simulink model "modelo_dp_completmod"  (Simulink 9.1)
settings: Solver=VariableStepDiscrete  StartTime=0.0  StopTime=sim_time  RelTol=1e-3  EnableMultiTasking=on
values from neighbouring files (symbols this model uses):
  control_fm_am = 1    [configura_modelo_dp_completmod.m]    (also in configura_modulador.m = 0; matlab_WS_mal.mat)
  f_cic_scale = ceil(log2((M*R)^(N-1)))    [conf_mod_filter_design.m]
  fc = 1    [configura_modelo_dp_completmod.m]    (also in configura_modulador.m; matlab_WS_mal.mat)
  fsc = 100    [configura_modelo_dp_completmod.m]    (also in configura_modulador.m; matlab_WS_mal.mat)
  h_comp_cic = round(h_comp_cic*2^16)*2^-16    [conf_mod_filter_design.m]
  h_comp_DAC = round(h_comp_DAC*2^17)*2^-17    [conf_mod_filter_design.m]
  Kfm = 5000    [configura_modelo_dp_completmod.m]    (also in configura_modulador.m; matlab_WS_mal.mat)
  L = 15    [conf_mod_filter_design.m]
  m_am = 1*(1-2^-15)    (= 0.999969482422)    [configura_modelo_dp_completmod.m]    (also in configura_modulador.m; matlab_WS_mal.mat)
  P = round(2^Macc*fmod*1e-3/(fsc/f_interpolacion))*2^-Macc    [conf_mod_filter_design.m]
  R = 2000    [conf_mod_filter_design.m]
  source_sel = 0    [configura_modelo_dp_completmod.m]    (also in configura_modulador.m; matlab_WS_mal.mat = 2)
  W = 16    [conf_mod_filter_design.m]
libraries: dspsigops x6, simulink x2
settings Model: Creator=jvalls  LastModifiedBy=jvalls
settings DataIOCC: LimitDataPoints=on
settings DebuggingCC: UnderspecifiedInitializationDetection=Simplified  MergeDetectMultiDrivingBlocksExec=error  SolverPrmCheckMsg=warning
settings GRTTargetCC: GeneratePreprocessorConditionals=Disable all  CombineOutputUpdateFcns=on  GRTInterface=off
settings ConfigComp: CovSFcnEnable=off

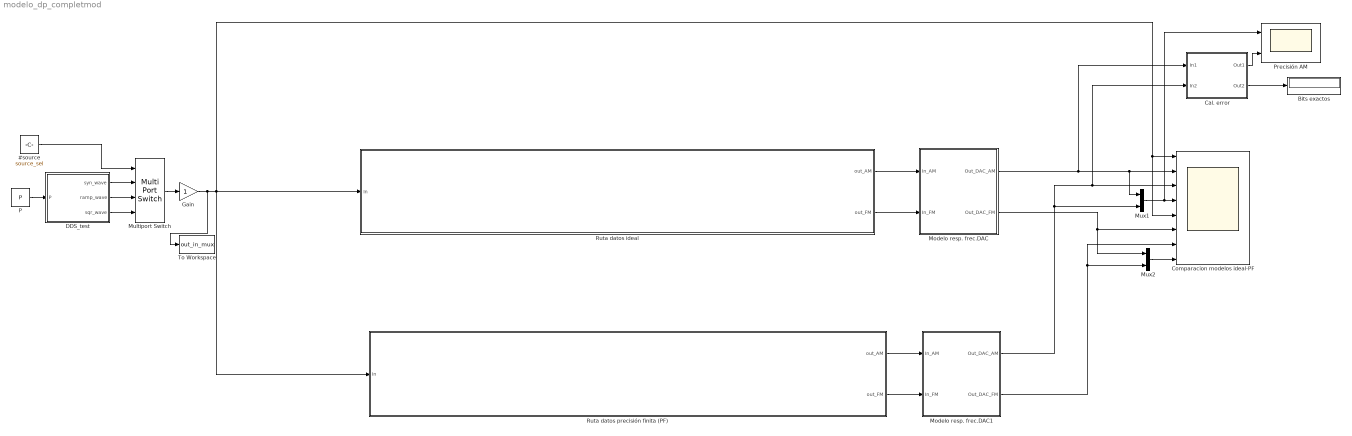
== system modelo_dp_completmod ==
  #source : Constant  Value=source_sel  SampleTime=R/fsc
  Bits exactos : Display
  Cal. error : Subsystem
  Comparacion modelos ideal-PF : Scope  NumInputPorts=8
  DDS_test : Subsystem
  Gain : Gain
  Modelo resp. frec.DAC : Subsystem
  Modelo resp. frec.DAC1 : Subsystem
  Multiport Switch : MultiPortSwitch  DataPortOrder=Specify indices  DataPortIndices={0,1,2}  OutDataTypeStr=double
  Mux1 : Mux  Inputs=2
  Mux2 : Mux  Inputs=2
  P : Constant  Value=P  OutDataTypeStr=fixdt(0,Macc,Macc)  SampleTime=R/fsc
  Precisión AM : Scope  NumInputPorts=2
  Ruta datos ideal : Subsystem
  Ruta datos precisión finita (PF) : Subsystem
  To Workspace : ToWorkspace  VariableName=out_in_mux  SampleTime=-1
      settings: Save2DSignal=2-D array (concatenate along first dimension)
  wires:
  Mux1/1 -> Precisión AM/1, Comparacion modelos ideal-PF/4
  Mux2/1 -> Comparacion modelos ideal-PF/8
  Modelo resp. frec.DAC/1(Out_DAC_AM) -> Cal. error/1(In1), Mux1/1, Comparacion modelos ideal-PF/2
  Modelo resp. frec.DAC1/1(Out_DAC_AM) -> Mux1/2, Cal. error/2(In2), Comparacion modelos ideal-PF/3
  Ruta datos ideal/1(out_AM) -> Modelo resp. frec.DAC/1(In_AM)
  Ruta datos precisión finita (PF)/1(out_AM) -> Modelo resp. frec.DAC1/1(In_AM)
  Ruta datos ideal/2(out_FM) -> Modelo resp. frec.DAC/2(In_FM)
  Ruta datos precisión finita (PF)/2(out_FM) -> Modelo resp. frec.DAC1/2(In_FM)
  Modelo resp. frec.DAC/2(Out_DAC_FM) -> Mux2/1, Comparacion modelos ideal-PF/6
  Modelo resp. frec.DAC1/2(Out_DAC_FM) -> Mux2/2, Comparacion modelos ideal-PF/7
  P/1 -> DDS_test/1(P)
  DDS_test/1(syn_wave) -> Multiport Switch/2
  DDS_test/2(ramp_wave) -> Multiport Switch/3
  DDS_test/3(sqr_wave) -> Multiport Switch/4
  #source/1 -> Multiport Switch/1
  Cal. error/1(Out1) -> Precisión AM/2
  Cal. error/2(Out2) -> Bits exactos/1
  Multiport Switch/1 -> Gain/1
  Gain/1 -> Comparacion modelos ideal-PF/5, Comparacion modelos ideal-PF/1, Ruta datos precisión finita (PF)/1(In), Ruta datos ideal/1(In), To Workspace/1

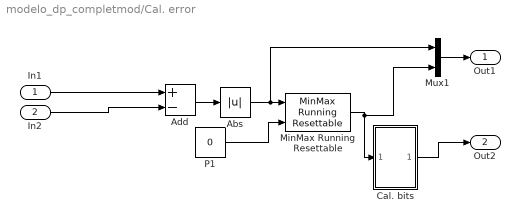
== system modelo_dp_completmod/Cal. error ==
  In1 : Inport
  In2 : Inport  Port=2
  Abs : Abs
  Add : Sum  Inputs=+-
  Cal. bits : Subsystem
  MinMax Running Resettable : simulink/Math Operations/MinMax Running Resettable  Function=max  vinit=0.0
  Mux1 : Mux  Inputs=2
  P1 : Constant  Value=0  OutDataTypeStr=double  SampleTime=-1
  Out1 : Outport
  Out2 : Outport  Port=2
  wires:
  In2/1 -> Add/2
  Abs/1 -> Mux1/1, MinMax Running Resettable/1
  MinMax Running Resettable/1 -> Mux1/2, Cal. bits/1(In1)
  In1/1 -> Add/1
  P1/1 -> MinMax Running Resettable/2
  Add/1 -> Abs/1
  Cal. bits/1(Out1) -> Out2/1
  Mux1/1 -> Out1/1

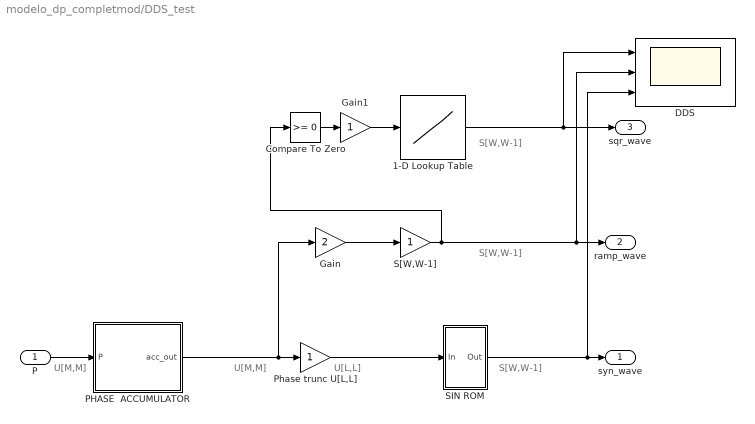
== system modelo_dp_completmod/DDS_test ==
  note: S[W,W-1]
  note: S[W,W-1]
  note: S[W,W-1]
  note: U[M,M]
  note: U[L,L]
  note: U[M,M]
  P : Inport
  1-D Lookup Table : Lookup_n-D  NumberOfTableDimensions=1  BreakpointsForDimension1=[0:1]  Table=[ -1+2^-(W-1) 1-2^-(W-1)]  InternalRulePriority=Speed  RndMeth=Simplest  InputSameDT=on
  Compare To Zero : simulink/Logic and Bit Operations/Compare To Zero  relop=>=  OutDataTypeStr=boolean
  DDS : Scope  NumInputPorts=3
  Gain : Gain  Gain=2  OutDataTypeStr=double
  Gain1 : Gain  OutDataTypeStr=double
  PHASE  ACCUMULATOR : Subsystem
  Phase trunc U[L,L] : Gain  OutDataTypeStr=fixdt(0,L,L)
  SIN ROM : Subsystem
  S[W,W-1] : Gain  OutDataTypeStr=fixdt(1,W,W-1)
  syn_wave : Outport
  ramp_wave : Outport  Port=2
  sqr_wave : Outport  Port=3
  wires:
  Phase trunc U[L,L]/1 -> SIN ROM/1(In)
  SIN ROM/1(Out) -> DDS/3, syn_wave/1
  P/1 -> PHASE  ACCUMULATOR/1(P)
  PHASE  ACCUMULATOR/1(acc_out) -> Phase trunc U[L,L]/1, Gain/1
  Gain1/1 -> 1-D Lookup Table/1
  Compare To Zero/1 -> Gain1/1
  1-D Lookup Table/1 -> sqr_wave/1, DDS/1
  S[W,W-1]/1 -> Compare To Zero/1, DDS/2, ramp_wave/1
  Gain/1 -> S[W,W-1]/1

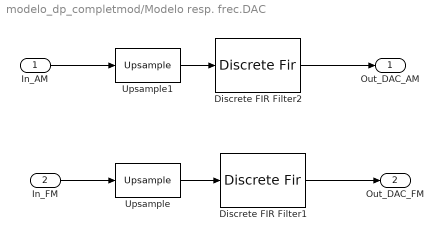
== system modelo_dp_completmod/Modelo resp. frec.DAC ==
  In_AM : Inport
  In_FM : Inport  Port=2
  Discrete FIR Filter1 : DiscreteFir  Coefficients=[1 1 1 1]  InputProcessing=Columns as channels (frame based)
  Discrete FIR Filter2 : DiscreteFir  Coefficients=[1 1 1 1]  InputProcessing=Columns as channels (frame based)
  Upsample : dspsigops/Upsample  N=4  phase=0  InputProcessing=Columns as channels (frame based)  RateOptions=Allow multirate processing  ic=0  mode=Unused parameter value
  Upsample1 : dspsigops/Upsample  N=4  phase=0  InputProcessing=Columns as channels (frame based)  RateOptions=Allow multirate processing  ic=0  mode=Unused parameter value
  Out_DAC_AM : Outport
  Out_DAC_FM : Outport  Port=2
  wires:
  Upsample1/1 -> Discrete FIR Filter2/1
  Upsample/1 -> Discrete FIR Filter1/1
  Discrete FIR Filter2/1 -> Out_DAC_AM/1
  In_AM/1 -> Upsample1/1
  In_FM/1 -> Upsample/1
  Discrete FIR Filter1/1 -> Out_DAC_FM/1

== system modelo_dp_completmod/Modelo resp. frec.DAC1 ==
  In_AM : Inport
  In_FM : Inport  Port=2
  Discrete FIR Filter1 : DiscreteFir  Coefficients=[1 1 1 1]  InputProcessing=Columns as channels (frame based)
  Discrete FIR Filter2 : DiscreteFir  Coefficients=[1 1 1 1]  InputProcessing=Columns as channels (frame based)
  Upsample : dspsigops/Upsample  N=4  phase=0  InputProcessing=Columns as channels (frame based)  RateOptions=Allow multirate processing  ic=0  mode=Unused parameter value
  Upsample1 : dspsigops/Upsample  N=4  phase=0  InputProcessing=Columns as channels (frame based)  RateOptions=Allow multirate processing  ic=0  mode=Unused parameter value
  Out_DAC_AM : Outport
  Out_DAC_FM : Outport  Port=2
  wires:
  Upsample1/1 -> Discrete FIR Filter2/1
  Upsample/1 -> Discrete FIR Filter1/1
  Discrete FIR Filter2/1 -> Out_DAC_AM/1
  In_AM/1 -> Upsample1/1
  In_FM/1 -> Upsample/1
  Discrete FIR Filter1/1 -> Out_DAC_FM/1

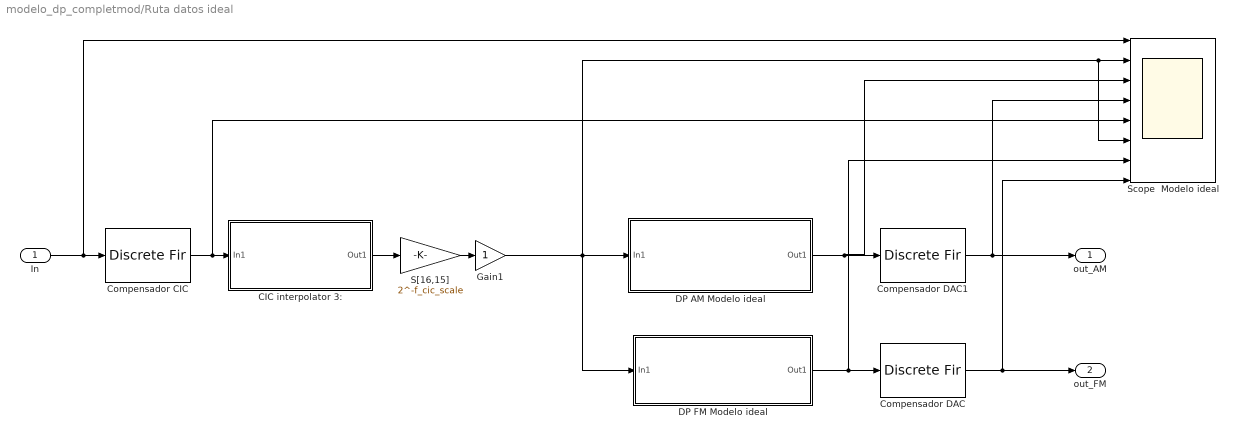
== system modelo_dp_completmod/Ruta datos ideal ==
  In : Inport
  "CIC interpolator 3: " : Subsystem
  Compensador CIC : DiscreteFir  Coefficients=h_comp_cic  InputProcessing=Columns as channels (frame based)
  Compensador DAC : DiscreteFir  Coefficients=h_comp_DAC  InputProcessing=Columns as channels (frame based)
  Compensador DAC1 : DiscreteFir  Coefficients=h_comp_DAC  InputProcessing=Columns as channels (frame based)
  DP AM Modelo ideal : Subsystem
  DP FM Modelo ideal : Subsystem
  Gain1 : Gain  OutDataTypeStr=double
  "S[16,15] " : Gain  Gain=2^-f_cic_scale  OutDataTypeStr=double
  Scope  Modelo ideal : Scope  NumInputPorts=8
  out_AM : Outport
  out_FM : Outport  Port=2
  wires:
  "CIC interpolator 3: "/1(Out1) -> "S[16,15] "/1
  "S[16,15] "/1 -> Gain1/1
  Gain1/1 -> Scope  Modelo ideal/6, Scope  Modelo ideal/2, DP AM Modelo ideal/1(In1), DP FM Modelo ideal/1(In1)
  DP FM Modelo ideal/1(Out1) -> Scope  Modelo ideal/7, Compensador DAC/1
  Compensador DAC/1 -> Scope  Modelo ideal/8, out_FM/1
  Compensador DAC1/1 -> out_AM/1, Scope  Modelo ideal/4
  Compensador CIC/1 -> Scope  Modelo ideal/5, "CIC interpolator 3: "/1(In1)
  DP AM Modelo ideal/1(Out1) -> Scope  Modelo ideal/3, Compensador DAC1/1
  In/1 -> Scope  Modelo ideal/1, Compensador CIC/1

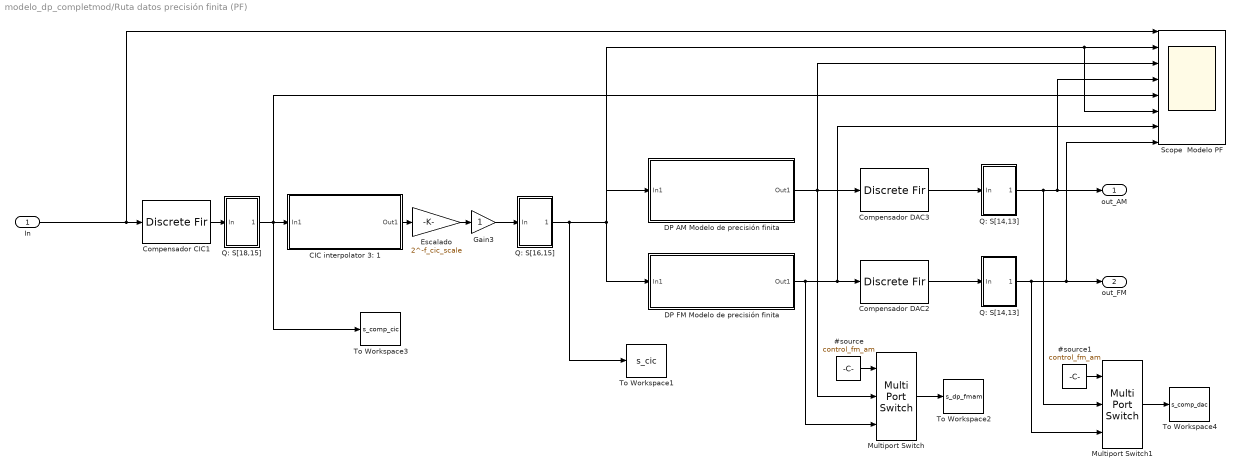
== system modelo_dp_completmod/Ruta datos precisión finita (PF) ==
  In : Inport
  #source : Constant  Value=control_fm_am  SampleTime=1/fsc
  #source1 : Constant  Value=control_fm_am  SampleTime=1/fsc
  CIC interpolator 3: 1 : Subsystem
  Compensador CIC1 : DiscreteFir  Coefficients=h_comp_cic  InputProcessing=Columns as channels (frame based)
  Compensador DAC2 : DiscreteFir  Coefficients=h_comp_DAC  InputProcessing=Columns as channels (frame based)
  Compensador DAC3 : DiscreteFir  Coefficients=h_comp_DAC  InputProcessing=Columns as channels (frame based)
  DP AM Modelo de precisión finita : Subsystem
  DP FM Modelo de precisión finita : Subsystem
  Escalado : Gain  Gain=2^-f_cic_scale  OutDataTypeStr=double
  Gain3 : Gain  OutDataTypeStr=double
  Multiport Switch : MultiPortSwitch  DataPortOrder=Specify indices  DataPortIndices={0,1}  OutDataTypeStr=double
  Multiport Switch1 : MultiPortSwitch  DataPortOrder=Specify indices  DataPortIndices={0,1}  OutDataTypeStr=double
  Q: S[14,13] : Subsystem
  "Q: S[14,13] " : Subsystem
  Q: S[16,15] : Subsystem
  Q: S[18,15] : Subsystem
  Scope  Modelo PF : Scope  NumInputPorts=8
  To Workspace1 : ToWorkspace  VariableName=s_cic  SampleTime=-1
      settings: Save2DSignal=2-D array (concatenate along first dimension)
  To Workspace2 : ToWorkspace  VariableName=s_dp_fmam  SampleTime=-1
      settings: Save2DSignal=2-D array (concatenate along first dimension)
  To Workspace3 : ToWorkspace  VariableName=s_comp_cic  SampleTime=-1
      settings: Save2DSignal=2-D array (concatenate along first dimension)
  To Workspace4 : ToWorkspace  VariableName=s_comp_dac  SampleTime=-1
      settings: Save2DSignal=2-D array (concatenate along first dimension)
  out_AM : Outport
  out_FM : Outport  Port=2
  wires:
  CIC interpolator 3: 1/1(Out1) -> Escalado/1
  Escalado/1 -> Gain3/1
  Compensador CIC1/1 -> Q: S[18,15]/1(In)
  Gain3/1 -> Q: S[16,15]/1(In)
  DP AM Modelo de precisión finita/1(Out1) -> Multiport Switch/2, Scope  Modelo PF/3, Compensador DAC3/1
  Compensador DAC2/1 -> "Q: S[14,13] "/1(In)
  DP FM Modelo de precisión finita/1(Out1) -> Multiport Switch/3, Scope  Modelo PF/7, Compensador DAC2/1
  Compensador DAC3/1 -> Q: S[14,13]/1(In)
  In/1 -> Scope  Modelo PF/1, Compensador CIC1/1
  Q: S[18,15]/1(Out1) -> To Workspace3/1, Scope  Modelo PF/5, CIC interpolator 3: 1/1(In1)
  Q: S[16,15]/1(Out1) -> To Workspace1/1, DP FM Modelo de precisión finita/1(In1), Scope  Modelo PF/6, Scope  Modelo PF/2, DP AM Modelo de precisión finita/1(In1)
  Multiport Switch/1 -> To Workspace2/1
  #source/1 -> Multiport Switch/1
  Q: S[14,13]/1(Out1) -> Multiport Switch1/2, out_AM/1, Scope  Modelo PF/4
  Multiport Switch1/1 -> To Workspace4/1
  #source1/1 -> Multiport Switch1/1
  "Q: S[14,13] "/1(Out1) -> Multiport Switch1/3, Scope  Modelo PF/8, out_FM/1

== system modelo_dp_completmod/Cal. error/Cal. bits ==
  In1 : Inport
  Divide : Product  Inputs=*/
  Math Function : Math  Operator=log10  SaturateOnIntegerOverflow=on
  Math Function1 : Math  Operator=log10  SaturateOnIntegerOverflow=on
  P2 : Constant  Value=2  OutDataTypeStr=double  SampleTime=-1
  Out1 : Outport
  wires:
  P2/1 -> Math Function1/1
  Math Function1/1 -> Divide/2
  In1/1 -> Math Function/1
  Math Function/1 -> Divide/1
  Divide/1 -> Out1/1

== system modelo_dp_completmod/DDS_test/PHASE  ACCUMULATOR ==
  P : Inport
  Add U[M,M] : Sum  AccumDataTypeStr=fixdt(0,Macc,Macc)  OutDataTypeStr=fixdt(0,24,24)  RndMeth=Convergent
  Delay2 : Delay  DelayLength=1  SampleTime=R/fsc
  acc_out : Outport
  wires:
  Add U[M,M]/1 -> acc_out/1, Delay2/1
  P/1 -> Add U[M,M]/2
  Delay2/1 -> Add U[M,M]/1

== system modelo_dp_completmod/DDS_test/SIN ROM ==
  In : Inport
  Add : Sum
  Constant : Constant  Value=2^-(L+1)  SampleTime=R/fsc
  Gain : Gain  Gain=2*pi
  Quantize LUT S[W,W-1] : Gain  OutDataTypeStr=fixdt(1,W,W-1)  RndMeth=Round  SaturateOnIntegerOverflow=on
  Saturation : Saturate  UpperLimit=1-2^-(W-1)  LowerLimit=-(1-2^-(W-1))
  Trigonometric Function1 : Trigonometry
  Out : Outport
  wires:
  Add/1 -> Gain/1
  In/1 -> Add/2
  Constant/1 -> Add/1
  Quantize LUT S[W,W-1]/1 -> Out/1
  Trigonometric Function1/1 -> Saturation/1
  Gain/1 -> Trigonometric Function1/1
  Saturation/1 -> Quantize LUT S[W,W-1]/1

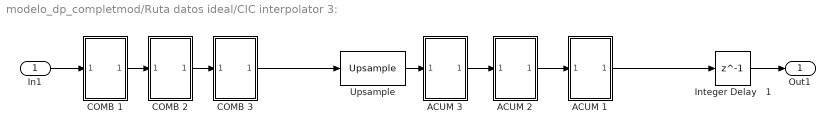
== system modelo_dp_completmod/Ruta datos ideal/CIC interpolator 3:  ==
  In1 : Inport
  "   Integer Delay   1" : Delay  DelayLength=1  InputProcessing=Inherited
  ACUM 1 : Subsystem
  ACUM 2 : Subsystem
  ACUM 3 : Subsystem
  COMB 1 : Subsystem
  COMB 2 : Subsystem
  COMB 3 : Subsystem
  Upsample : dspsigops/Upsample  N=R  phase=0  InputProcessing=Columns as channels (frame based)  RateOptions=Allow multirate processing  ic=0  mode=Unused parameter value
  Out1 : Outport
  wires:
  "   Integer Delay   1"/1 -> Out1/1
  In1/1 -> COMB 1/1(In1)
  COMB 1/1(Out1) -> COMB 2/1(In1)
  COMB 2/1(Out1) -> COMB 3/1(In1)
  ACUM 2/1(Out1) -> ACUM 1/1(In1)
  Upsample/1 -> ACUM 3/1(In1)
  ACUM 3/1(Out1) -> ACUM 2/1(In1)
  ACUM 1/1(Out1) -> "   Integer Delay   1"/1
  COMB 3/1(Out1) -> Upsample/1

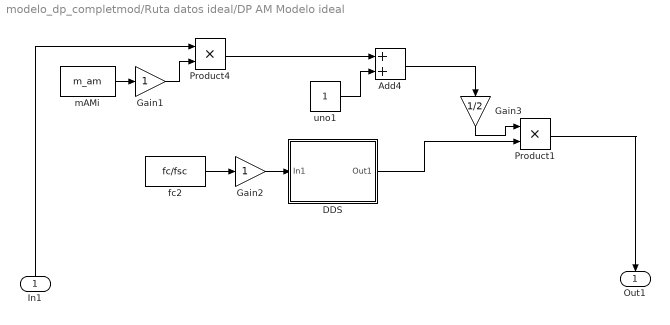
== system modelo_dp_completmod/Ruta datos ideal/DP AM Modelo ideal ==
  In1 : Inport
  Add4 : Sum
  DDS : Subsystem
  Gain1 : Gain  OutDataTypeStr=double
  Gain2 : Gain  OutDataTypeStr=double
  Gain3 : Gain  Gain=1/2  OutDataTypeStr=double
  Product1 : Product
  Product4 : Product
  fc2 : Constant  Value=fc/fsc  OutDataTypeStr=fixdt(0,24,24)
  "mAMi " : Constant  Value=m_am  OutDataTypeStr=fixdt(0,16,15)
  uno1 : Constant
  Out1 : Outport
  wires:
  Product1/1 -> Out1/1
  Gain3/1 -> Product1/1
  In1/1 -> Product4/1
  Add4/1 -> Gain3/1
  uno1/1 -> Add4/2
  Product4/1 -> Add4/1
  "mAMi "/1 -> Gain1/1
  DDS/1(Out1) -> Product1/2
  fc2/1 -> Gain2/1
  Gain1/1 -> Product4/2
  Gain2/1 -> DDS/1(In1)

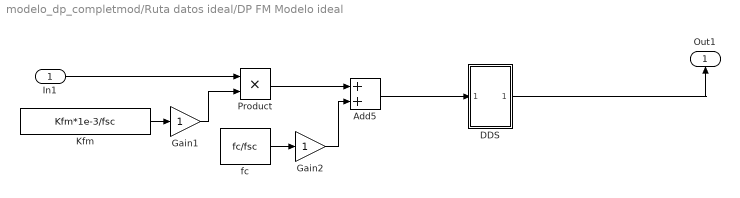
== system modelo_dp_completmod/Ruta datos ideal/DP FM Modelo ideal ==
  In1 : Inport
  Add5 : Sum
  DDS : Subsystem
  Gain1 : Gain  OutDataTypeStr=double
  Gain2 : Gain  OutDataTypeStr=double
  Kfm : Constant  Value=Kfm*1e-3/fsc  OutDataTypeStr=fixdt(0,16,16)
  Product : Product
  fc : Constant  Value=fc/fsc  OutDataTypeStr=fixdt(0,24,24)
  Out1 : Outport
  wires:
  DDS/1(Out1) -> Out1/1
  Add5/1 -> DDS/1(In1)
  Product/1 -> Add5/1
  In1/1 -> Product/1
  fc/1 -> Gain2/1
  Kfm/1 -> Gain1/1
  Gain1/1 -> Product/2
  Gain2/1 -> Add5/2

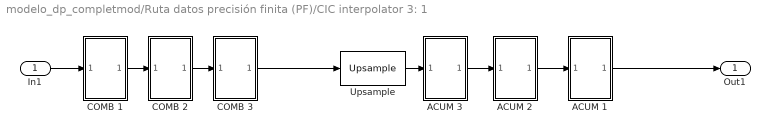
== system modelo_dp_completmod/Ruta datos precisión finita (PF)/CIC interpolator 3: 1 ==
  In1 : Inport
  ACUM 1 : Subsystem
  ACUM 2 : Subsystem
  ACUM 3 : Subsystem
  COMB 1 : Subsystem
  COMB 2 : Subsystem
  COMB 3 : Subsystem
  Upsample : dspsigops/Upsample  N=R  phase=0  InputProcessing=Columns as channels (frame based)  RateOptions=Allow multirate processing  ic=0  mode=Unused parameter value
  Out1 : Outport
  wires:
  ACUM 1/1(Out1) -> Out1/1
  In1/1 -> COMB 1/1(In1)
  COMB 1/1(Out1) -> COMB 2/1(In1)
  COMB 2/1(Out1) -> COMB 3/1(In1)
  ACUM 2/1(Out1) -> ACUM 1/1(In1)
  Upsample/1 -> ACUM 3/1(In1)
  ACUM 3/1(Out1) -> ACUM 2/1(In1)
  COMB 3/1(Out1) -> Upsample/1

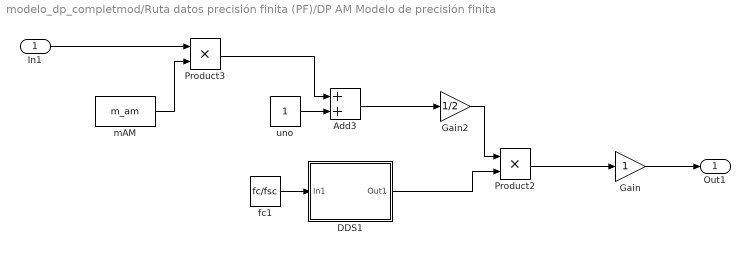
== system modelo_dp_completmod/Ruta datos precisión finita (PF)/DP AM Modelo de precisión finita ==
  In1 : Inport
  Add3 : Sum  AccumDataTypeStr=fixdt(1,17,15)
  DDS1 : Subsystem
  Gain : Gain  OutDataTypeStr=double
  Gain2 : Gain  Gain=1/2  OutDataTypeStr=fixdt(1,17,15)
  Product2 : Product  OutDataTypeStr=fixdt(1,16,15)
  Product3 : Product  OutDataTypeStr=fixdt(1,16,15)
  fc1 : Constant  Value=fc/fsc  OutDataTypeStr=fixdt(0,24,24)
  mAM : Constant  Value=m_am  OutDataTypeStr=fixdt(0,16,15)
  uno : Constant  OutDataTypeStr=fixdt(0,16,15)
  Out1 : Outport
  wires:
  uno/1 -> Add3/2
  Gain/1 -> Out1/1
  Product2/1 -> Gain/1
  Add3/1 -> Gain2/1
  Product3/1 -> Add3/1
  DDS1/1(Out1) -> Product2/2
  mAM/1 -> Product3/2
  In1/1 -> Product3/1
  fc1/1 -> DDS1/1(In1)
  Gain2/1 -> Product2/1

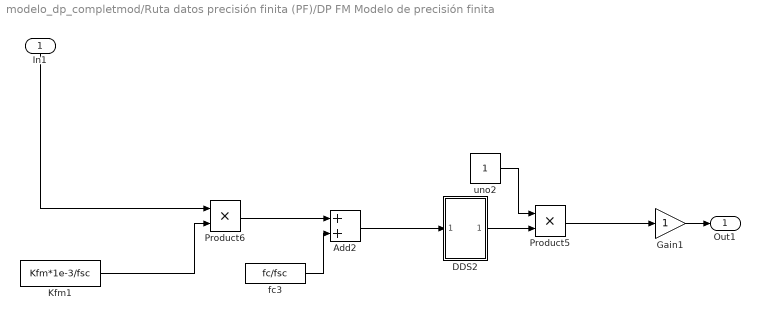
== system modelo_dp_completmod/Ruta datos precisión finita (PF)/DP FM Modelo de precisión finita ==
  In1 : Inport
  Add2 : Sum  AccumDataTypeStr=double  OutDataTypeStr=fixdt(1,24,24)
  DDS2 : Subsystem
  Gain1 : Gain  OutDataTypeStr=double
  Kfm1 : Constant  Value=Kfm*1e-3/fsc  OutDataTypeStr=fixdt(0,16,16)
  Product5 : Product  OutDataTypeStr=fixdt(1,16,15)
  Product6 : Product  OutDataTypeStr=fixdt(1,24,24)
  fc3 : Constant  Value=fc/fsc  OutDataTypeStr=fixdt(0,24,24)
  uno2 : Constant  OutDataTypeStr=fixdt(0,17,15)
  Out1 : Outport
  wires:
  Product6/1 -> Add2/1
  fc3/1 -> Add2/2
  In1/1 -> Product6/1
  uno2/1 -> Product5/1
  DDS2/1(Out1) -> Product5/2
  Kfm1/1 -> Product6/2
  Gain1/1 -> Out1/1
  Product5/1 -> Gain1/1
  Add2/1 -> DDS2/1(In1)

== system modelo_dp_completmod/Ruta datos precisión finita (PF)/Q: S[14,13] ==
  In : Inport
  Gain : Gain  OutDataTypeStr=double
  S[14,13] floor : Gain  OutDataTypeStr=fixdt(1,14,13)
  Out1 : Outport
  wires:
  In/1 -> S[14,13] floor/1
  S[14,13] floor/1 -> Gain/1
  Gain/1 -> Out1/1

== system modelo_dp_completmod/Ruta datos precisión finita (PF)/Q: S[14,13]  ==
  In : Inport
  Gain : Gain  OutDataTypeStr=double
  S[14,13] floor : Gain  OutDataTypeStr=fixdt(1,14,13)
  Out1 : Outport
  wires:
  In/1 -> S[14,13] floor/1
  S[14,13] floor/1 -> Gain/1
  Gain/1 -> Out1/1

== system modelo_dp_completmod/Ruta datos precisión finita (PF)/Q: S[16,15] ==
  In : Inport
  Gain : Gain  OutDataTypeStr=double
  S[16,15] floor : Gain  OutDataTypeStr=fixdt(1,16,15)
  Out1 : Outport
  wires:
  In/1 -> S[16,15] floor/1
  S[16,15] floor/1 -> Gain/1
  Gain/1 -> Out1/1

== system modelo_dp_completmod/Ruta datos precisión finita (PF)/Q: S[18,15] ==
  In : Inport
  Gain : Gain  OutDataTypeStr=double
  S[18,15] floor : Gain  OutDataTypeStr=fixdt(1,18,15)
  Out1 : Outport
  wires:
  In/1 -> S[18,15] floor/1
  S[18,15] floor/1 -> Gain/1
  Gain/1 -> Out1/1

== system modelo_dp_completmod/Ruta datos ideal/CIC interpolator 3: /ACUM 1 ==
  In1 : Inport
  "   Integer Delay   " : Delay  DelayLength=1  InputProcessing=Inherited
  Add11 : Sum
  Out1 : Outport
  wires:
  In1/1 -> Add11/2
  "   Integer Delay   "/1 -> Out1/1, Add11/1
  Add11/1 -> "   Integer Delay   "/1

== system modelo_dp_completmod/Ruta datos ideal/CIC interpolator 3: /ACUM 2 ==
  In1 : Inport
  "   Integer Delay   " : Delay  DelayLength=1  InputProcessing=Inherited
  Add11 : Sum
  Out1 : Outport
  wires:
  In1/1 -> Add11/2
  "   Integer Delay   "/1 -> Out1/1, Add11/1
  Add11/1 -> "   Integer Delay   "/1

== system modelo_dp_completmod/Ruta datos ideal/CIC interpolator 3: /ACUM 3 ==
  In1 : Inport
  "   Integer Delay   " : Delay  DelayLength=1  InputProcessing=Inherited
  Add11 : Sum
  Out1 : Outport
  wires:
  In1/1 -> Add11/2
  "   Integer Delay   "/1 -> Out1/1, Add11/1
  Add11/1 -> "   Integer Delay   "/1

== system modelo_dp_completmod/Ruta datos ideal/CIC interpolator 3: /COMB 1 ==
  In1 : Inport
  Add8 : Sum  Inputs=+-
  "Integer Delay " : Delay  DelayLength=1  InputProcessing=Inherited
  Out1 : Outport
  wires:
  Add8/1 -> Out1/1
  In1/1 -> "Integer Delay "/1, Add8/1
  "Integer Delay "/1 -> Add8/2

== system modelo_dp_completmod/Ruta datos ideal/CIC interpolator 3: /COMB 2 ==
  In1 : Inport
  Add8 : Sum  Inputs=+-
  "Integer Delay " : Delay  DelayLength=1  InputProcessing=Inherited
  Out1 : Outport
  wires:
  Add8/1 -> Out1/1
  In1/1 -> "Integer Delay "/1, Add8/1
  "Integer Delay "/1 -> Add8/2

== system modelo_dp_completmod/Ruta datos ideal/CIC interpolator 3: /COMB 3 ==
  In1 : Inport
  Add8 : Sum  Inputs=+-
  "Integer Delay " : Delay  DelayLength=1  InputProcessing=Inherited
  Out1 : Outport
  wires:
  Add8/1 -> Out1/1
  In1/1 -> "Integer Delay "/1, Add8/1
  "Integer Delay "/1 -> Add8/2

== system modelo_dp_completmod/Ruta datos ideal/DP AM Modelo ideal/DDS ==
  In1 : Inport
  Add1 : Sum
  Add6 : Sum
  Delay1 : Delay  DelayLength=1
  Gain : Gain  Gain=2*pi
  Trigonometric Function1 : Trigonometry
  fc4 : Constant  Value=2*pi*2^-(15+1)
  Out1 : Outport
  wires:
  Trigonometric Function1/1 -> Out1/1
  Add6/1 -> Trigonometric Function1/1
  Add1/1 -> Delay1/1, Gain/1
  In1/1 -> Add1/2
  fc4/1 -> Add6/2
  Gain/1 -> Add6/1
  Delay1/1 -> Add1/1

== system modelo_dp_completmod/Ruta datos ideal/DP FM Modelo ideal/DDS ==
  In1 : Inport
  Add : Sum
  Add7 : Sum
  Delay : Delay  DelayLength=1
  Gain : Gain  Gain=2*pi
  Trigonometric Function : Trigonometry
  fc5 : Constant  Value=2*pi*2^-(15+1)
  Out1 : Outport
  wires:
  Trigonometric Function/1 -> Out1/1
  fc5/1 -> Add7/2
  In1/1 -> Add/2
  Add/1 -> Gain/1, Delay/1
  Add7/1 -> Trigonometric Function/1
  Gain/1 -> Add7/1
  Delay/1 -> Add/1

== system modelo_dp_completmod/Ruta datos precisión finita (PF)/CIC interpolator 3: 1/ACUM 1 ==
  In1 : Inport
  "   Integer Delay   " : Delay  DelayLength=1  InputProcessing=Inherited
  Add11 : Sum
  Out1 : Outport
  wires:
  In1/1 -> Add11/2
  Add11/1 -> Out1/1, "   Integer Delay   "/1
  "   Integer Delay   "/1 -> Add11/1

== system modelo_dp_completmod/Ruta datos precisión finita (PF)/CIC interpolator 3: 1/ACUM 2 ==
  In1 : Inport
  "   Integer Delay   " : Delay  DelayLength=1  InputProcessing=Inherited
  Add11 : Sum
  Out1 : Outport
  wires:
  In1/1 -> Add11/2
  Add11/1 -> Out1/1, "   Integer Delay   "/1
  "   Integer Delay   "/1 -> Add11/1

== system modelo_dp_completmod/Ruta datos precisión finita (PF)/CIC interpolator 3: 1/ACUM 3 ==
  In1 : Inport
  "   Integer Delay   " : Delay  DelayLength=1  InputProcessing=Inherited
  Add11 : Sum
  Out1 : Outport
  wires:
  In1/1 -> Add11/2
  Add11/1 -> Out1/1, "   Integer Delay   "/1
  "   Integer Delay   "/1 -> Add11/1

== system modelo_dp_completmod/Ruta datos precisión finita (PF)/CIC interpolator 3: 1/COMB 1 ==
  In1 : Inport
  Add8 : Sum  Inputs=+-
  "Integer Delay " : Delay  DelayLength=1  InputProcessing=Inherited
  Out1 : Outport
  wires:
  Add8/1 -> Out1/1
  In1/1 -> "Integer Delay "/1, Add8/1
  "Integer Delay "/1 -> Add8/2

== system modelo_dp_completmod/Ruta datos precisión finita (PF)/CIC interpolator 3: 1/COMB 2 ==
  In1 : Inport
  Add8 : Sum  Inputs=+-
  "Integer Delay " : Delay  DelayLength=1  InputProcessing=Inherited
  Out1 : Outport
  wires:
  Add8/1 -> Out1/1
  In1/1 -> "Integer Delay "/1, Add8/1
  "Integer Delay "/1 -> Add8/2

== system modelo_dp_completmod/Ruta datos precisión finita (PF)/CIC interpolator 3: 1/COMB 3 ==
  In1 : Inport
  Add8 : Sum  Inputs=+-
  "Integer Delay " : Delay  DelayLength=1  InputProcessing=Inherited
  Out1 : Outport
  wires:
  Add8/1 -> Out1/1
  In1/1 -> "Integer Delay "/1, Add8/1
  "Integer Delay "/1 -> Add8/2

== system modelo_dp_completmod/Ruta datos precisión finita (PF)/DP AM Modelo de precisión finita/DDS1 ==
  In1 : Inport
  Add2 : Sum  AccumDataTypeStr=fixdt(0,24,24)  OutDataTypeStr=fixdt(0,24,24)  RndMeth=Convergent
  Delay4 : Delay  DelayLength=1
  Gain1 : Gain  OutDataTypeStr=double
  Phase trunc : Gain  OutDataTypeStr=fixdt(0,15,15)
  SIN ROM : Subsystem
  Out1 : Outport
  wires:
  Add2/1 -> Gain1/1
  Phase trunc/1 -> SIN ROM/1(In1)
  In1/1 -> Add2/2
  SIN ROM/1(Out1) -> Out1/1
  Gain1/1 -> Delay4/1, Phase trunc/1
  Delay4/1 -> Add2/1

== system modelo_dp_completmod/Ruta datos precisión finita (PF)/DP FM Modelo de precisión finita/DDS2 ==
  In1 : Inport
  Add8 : Sum  AccumDataTypeStr=fixdt(0,24,24)  OutDataTypeStr=fixdt(0,24,24)  RndMeth=Convergent
  Delay2 : Delay  DelayLength=1
  Phase trunc : Gain  OutDataTypeStr=fixdt(0,15,15)
  SIN ROM : Subsystem
  Out1 : Outport
  wires:
  Phase trunc/1 -> SIN ROM/1(In1)
  Add8/1 -> Phase trunc/1, Delay2/1
  SIN ROM/1(Out1) -> Out1/1
  In1/1 -> Add8/2
  Delay2/1 -> Add8/1

== system modelo_dp_completmod/Ruta datos precisión finita (PF)/DP AM Modelo de precisión finita/DDS1/SIN ROM ==
  In1 : Inport
  Add : Sum
  Constant : Constant  Value=2^-(15+1)
  Gain : Gain  Gain=2*pi
  Gain1 : Gain  OutDataTypeStr=fixdt(1,16,15)  RndMeth=Round  SaturateOnIntegerOverflow=on
  Trigonometric Function1 : Trigonometry
  Out1 : Outport
  wires:
  Add/1 -> Gain/1
  In1/1 -> Add/2
  Constant/1 -> Add/1
  Gain1/1 -> Out1/1
  Trigonometric Function1/1 -> Gain1/1
  Gain/1 -> Trigonometric Function1/1

== system modelo_dp_completmod/Ruta datos precisión finita (PF)/DP FM Modelo de precisión finita/DDS2/SIN ROM ==
  In1 : Inport
  Add : Sum
  Constant : Constant  Value=2^-(15+1)
  Gain : Gain  Gain=2*pi
  Gain1 : Gain  OutDataTypeStr=fixdt(1,16,15)  RndMeth=Round  SaturateOnIntegerOverflow=on
  Saturation : Saturate  UpperLimit=1-2^-15  LowerLimit=-(1-2^-15)
  Trigonometric Function1 : Trigonometry
  Out1 : Outport
  wires:
  Add/1 -> Gain/1
  In1/1 -> Add/2
  Constant/1 -> Add/1
  Gain1/1 -> Out1/1
  Trigonometric Function1/1 -> Saturation/1
  Gain/1 -> Trigonometric Function1/1
  Saturation/1 -> Gain1/1
